simulink model "States3"  (R2020a)
settings: Solver=FixedStepDiscrete  StartTime=0.0  StopTime=0.2  FixedStep=0.1  RelTol=1e-3  EnableMultiTasking=on
settings Model: Creator=bzhan  LastModifiedBy=bzhan
settings SolverCC: AutoInsertRateTranBlk=on
settings DataIOCC: LimitDataPoints=on
settings OptimizationCC: LifeSpan=inf
settings DebuggingCC: AllowSymbolicDim=off  SFUnexpectedBacktrackingDiag=warning  SFNoUnconditionalDefaultTransitionDiag=warning  SFExecutionAtInitializationDiag=none  ArithmeticOperatorsInVariantConditions=warning
settings SFSimCC: SimUseLocalCustomCode=off  CustomCodeUndefinedFunction=UseInterfaceOnly
settings RTWCC: RTWUseLocalCustomCode=off
settings CodeAppCC: StateflowObjectComments=on
settings GRTTargetCC: TargetLangStandard=C89/C90 (ANSI)
settings ConfigComp: CovMetricSettings=dw  CovHtmlReporting=on  CovSaveCumulativeToWorkspaceVar=on  CovSaveSingleToWorkspaceVar=on  CovShowResultsExplorer=off  CovExternalEMLEnable=off  CovSFcnEnable=off

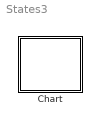
== system States3 ==
  Chart : Stateflow chart  TreatAsAtomicUnit=on

== stateflow chart States3/Chart ==
  settings: updateMethod=DISCRETE  sampleTime=0.1
  state A
    en: f("enA")
    ex: f("exA")
    state A1 [parallel]
      en: f("enA1")
      ex: f("exA1")
      settings: executionOrder=1
    state A2 [parallel]
      en: f("enA2")
      ex: f("exA2")
      settings: executionOrder=2
  state B
    en: f("enB")
    du: f("duB")
    ex: f("exB")
    state B1 [parallel]
      en: f("enB1")
      du: f("duB1")
      ex: f("exB1")
      settings: executionOrder=1
    state B2 [parallel]
      en: f("enB2")
      du: f("duB2")
      ex: f("exB2")
      settings: executionOrder=2
  (default) -> A
  A -> B
  data: s function_input
  function f(s):
    | function f(s)
    |   fprintf(s+"\n");
